simulink model "tankcontrol_nonlin_model_PI_controller_control101"  (R2025b)
settings: Solver=VariableStepAuto  StartTime=0.0  StopTime=300  RelTol=1e-3
undefined symbols (not defined in the file or in its folder): beta1rel, beta2rel, gamma1rel, gamma2rel, h10rel, h20rel, u0
settings Model: Creator=barsr  LastModifiedBy=barsr
settings RTWCC: GPUComputeCapability=3.5

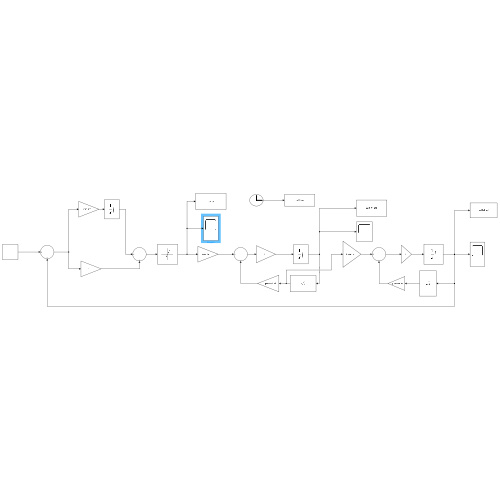
[thumbnail: Simulink's stored preview of the top-level diagram]
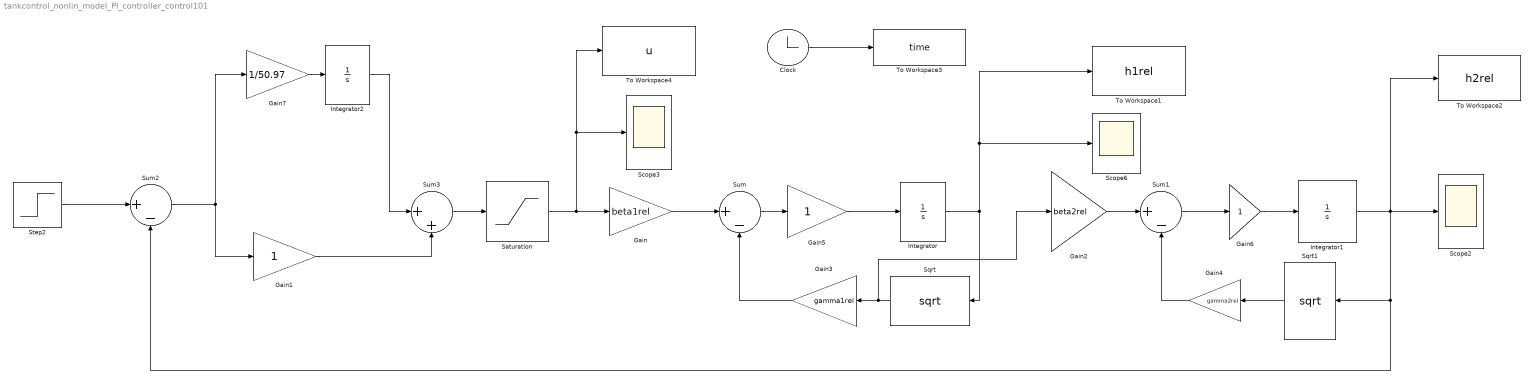
== system tankcontrol_nonlin_model_PI_controller_control101 ==
  Clock : Clock
  Gain : Gain  Gain=beta1rel
  Gain1 : Gain
  Gain2 : Gain  Gain=beta2rel
  Gain3 : Gain  Gain=gamma1rel
  Gain4 : Gain  Gain=gamma2rel
  Gain5 : Gain
  Gain6 : Gain
  Gain7 : Gain  Gain=1/50.97
  Integrator : Integrator  InitialCondition=h10rel  LimitOutput=on  UpperSaturationLimit=1  LowerSaturationLimit=0
  Integrator1 : Integrator  InitialCondition=h20rel  LimitOutput=on  UpperSaturationLimit=1  LowerSaturationLimit=0
  Integrator2 : Integrator  InitialCondition=u0  LimitOutput=on  UpperSaturationLimit=1  LowerSaturationLimit=0
  Saturation : Saturate  UpperLimit=1  LowerLimit=0
  Scope2 : Scope
      settings: ActiveDisplayYMinimum=-0.76866162703230412  ActiveDisplayYMaximum=1.4291405570926656
  Scope3 : Scope
      settings: ActiveDisplayYMinimum=-1.9782110778290463  ActiveDisplayYMaximum=3.1066207786599094
  Scope6 : Scope
      settings: ActiveDisplayYMinimum=0.047832795682999862  ActiveDisplayYMaximum=0.46548620585467054  DataLoggingVariableName=ScopeData4
  Sqrt : Sqrt
  Sqrt1 : Sqrt
  Step2 : Step  Time=0  Before=0.6371  After=0.9371  SampleTime=0
  Sum : Sum  Inputs=|+-
  Sum1 : Sum  Inputs=|+-
  Sum2 : Sum  Inputs=|+-
  Sum3 : Sum  Inputs=|++
  To Workspace1 : ToWorkspace  VariableName=h1rel  SampleTime=-1
  To Workspace2 : ToWorkspace  VariableName=h2rel  SampleTime=-1
  To Workspace3 : ToWorkspace  VariableName=time  SampleTime=-1
  To Workspace4 : ToWorkspace  VariableName=u  SampleTime=-1
  wires:
  Gain/1 -> Sum/1
  Sum/1 -> Gain5/1
  Sum1/1 -> Gain6/1
  Gain5/1 -> Integrator/1
  Gain6/1 -> Integrator1/1
  Gain4/1 -> Sum1/2
  Clock/1 -> To Workspace3/1
  Step2/1 -> Sum2/1
  Saturation/1 -> To Workspace4/1, Scope3/1, Gain/1
  Gain2/1 -> Sum1/1
  Integrator/1 -> Scope6/1, To Workspace1/1, Sqrt/1
  Gain3/1 -> Sum/2
  Sqrt/1 -> Gain2/1, Gain3/1
  Sqrt1/1 -> Gain4/1
  Integrator1/1 -> To Workspace2/1, Sqrt1/1, Sum2/2, Scope2/1
  Sum2/1 -> Gain1/1, Gain7/1
  Gain7/1 -> Integrator2/1
  Integrator2/1 -> Sum3/1
  Gain1/1 -> Sum3/2
  Sum3/1 -> Saturation/1
